simulink model "Top_Model"  (R2020a)
settings: Solver=ode4  StartTime=0.0  StopTime=60  FixedStep=DT  MaxStep=DT  RelTol=1e-3  EnableMultiTasking=on
values from neighbouring files (symbols this model uses):
  OutList = get_OutList(outfile_path)    [run_Top_Model_multi.m]
  tp = turbine_params_5MW()    [baseline_design.m]    (also in run_Top_Model.m)
undefined symbols (not defined in the file or in its folder): strmatch
settings Model: Creator=bjonkman  LastModifiedBy=lpwoolcock
settings SolverCC: AutoInsertRateTranBlk=on
settings DataIOCC: SaveFormat=Array  SignalLoggingSaveFormat=ModelDataLogs  SaveOutput=off  SaveTime=off  ReturnWorkspaceOutputs=off  SignalLoggingName=sigsOut
settings OptimizationCC: ExpressionDepthLimit=2147483647  LifeSpan=inf
settings DebuggingCC: SaveWithParameterizedLinksMsg=none  UnderspecifiedInitializationDetection=Classic  MergeDetectMultiDrivingBlocksExec=none  SignalResolutionControl=TryResolveAllWithWarning  MultiTaskDSMMsg=warning  MultiTaskCondExecSysMsg=none  FcnCallInpInsideContextMsg=warning  StateNameClashWarn=warning  SFUnexpectedBacktrackingDiag=warning  SFNoUnconditionalDefaultTransitionDiag=warning  SFExecutionAtInitializationDiag=none  ArithmeticOperatorsInVariantConditions=warning
settings HardwareCC: ProdBitPerPointer=32  ProdBitPerSizeT=32  ProdBitPerPtrDiffT=32  ProdLargestAtomicFloat=None  ProdIntDivRoundTo=Undefined  ProdEndianess=Unspecified  ProdWordSize=32  ProdHWDeviceType=32-bit Generic  TargetUnknown=on
settings ModelReferenceCC: PropagateSignalLabelsOutOfModel=off
settings SFSimCC: SimUseLocalCustomCode=off  CustomCodeUndefinedFunction=UseInterfaceOnly
settings RTWCC: RTWUseLocalCustomCode=off
settings CodeAppCC: StateflowObjectComments=on
settings GRTTargetCC: TargetLangStandard=C89/C90 (ANSI)  ModelReferenceCompliant=off  ParMdlRefBuildCompliant=off  CompOptLevelCompliant=off  ConcurrentExecutionCompliant=off  CombineOutputUpdateFcns=off  MatFileLogging=off  GRTInterface=on
settings ConfigComp: CovMetricSettings=dw  CovHtmlReporting=on  CovSaveCumulativeToWorkspaceVar=on  CovSaveSingleToWorkspaceVar=on  CovExternalEMLEnable=off

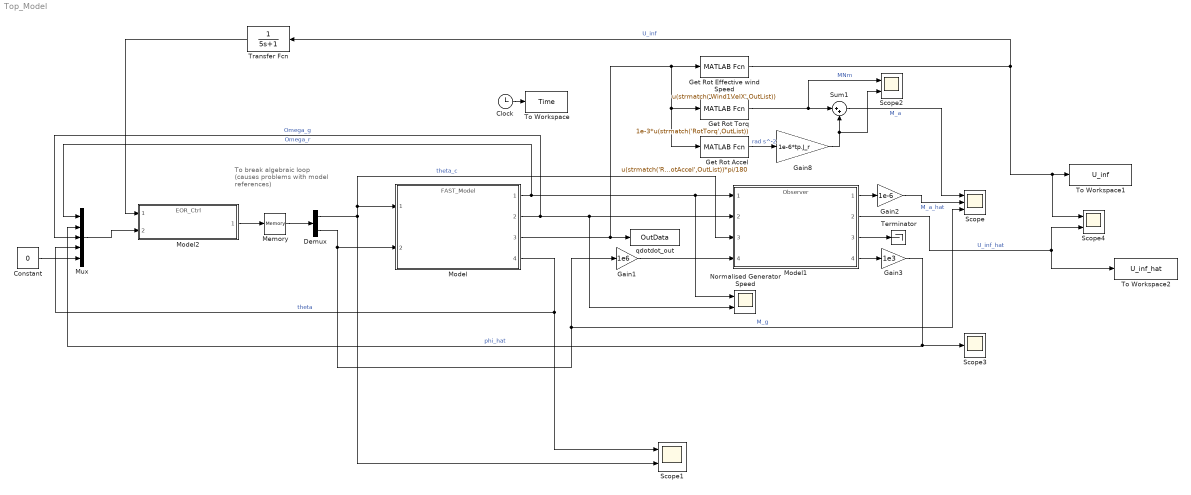
== system Top_Model ==
  note: To break algebraic loop (causes problems with model references)
  Clock : Clock
  Constant : Constant  Value=0
  Demux : Demux  Outputs=2
  Gain1 : Gain  Gain=1e6
  Gain2 : Gain  Gain=1e-6
  Gain3 : Gain  Gain=1e3
  Gain8 : Gain  Gain=1e-6*tp.J_r
  Get Rot Accel : MATLABFcn  MATLABFcn=u(strmatch('RotAccel',OutList))*pi/180
  Get Rot Effective wind Speed : MATLABFcn  MATLABFcn=u(strmatch('Wind1VelX',OutList))
  Get Rot Torq : MATLABFcn  MATLABFcn=1e-3*u(strmatch('RotTorq',OutList))
  Memory : Memory
  Model : ModelReference  ModelNameDialog=FAST_Model.slx  SimulationMode=Normal  ModelReferenceVersion=1.8
  Model1 : ModelReference  ModelNameDialog=Observer.slx  SimulationMode=Normal  ModelReferenceVersion=1.15
  Model2 : ModelReference  ModelNameDialog=EOR_Ctrl.slx  SimulationMode=Normal  ModelReferenceVersion=1.66
  Mux : Mux  Inputs=5
  Normalised Generator Speed : Scope  NumInputPorts=2
  Scope : Scope  NumInputPorts=3
  Scope1 : Scope  NumInputPorts=2
  Scope2 : Scope  NumInputPorts=2
  Scope3 : Scope
  Scope4 : Scope  NumInputPorts=2
  Sum1 : Sum  Inputs=|++
  Terminator : Terminator
  To Workspace : ToWorkspace  VariableName=Time  SampleTime=-1
  To Workspace1 : ToWorkspace  VariableName=U_inf  SaveFormat=Timeseries  SampleTime=-1
  To Workspace2 : ToWorkspace  VariableName=U_inf_hat  SaveFormat=Timeseries  SampleTime=-1
  Transfer Fcn : TransferFcn  Denominator=[5 1]
  qdotdot_out : ToWorkspace  VariableName=OutData  SampleTime=-1
  wires:
  Clock/1 -> To Workspace/1
  Model/3 -> Get Rot Accel/1, Get Rot Torq/1, Get Rot Effective wind Speed/1, qdotdot_out/1
  Get Rot Effective wind Speed/1 -> To Workspace1/1, Scope4/1, Transfer Fcn/1  "U_inf"
  Model1/1 -> Gain2/1
  Get Rot Accel/1 -> Gain8/1  "rad s^-2"
  Get Rot Torq/1 -> Scope2/1, Sum1/1  "MNm"
  Sum1/1 -> Scope/1  "M_a"
  Gain8/1 -> Sum1/2, Scope2/2
  Model/1 -> Mux/1, Normalised Generator Speed/1, Model1/1  "Omega_r"
  Model/2 -> Mux/3, Model1/2, Normalised Generator Speed/2  "Omega_g"
  Model1/3 -> Terminator/1
  Model/4 -> Mux/4, Scope1/1  "theta"
  Model2/1 -> Memory/1
  Memory/1 -> Demux/1
  Mux/1 -> Model2/2
  Model1/4 -> Gain3/1
  Constant/1 -> Mux/5
  Demux/1 -> Model1/3, Model/1, Scope1/2  "theta_c"
  Demux/2 -> Model/2, Gain1/1, Scope/3  "M_g"
  Gain1/1 -> Model1/4
  Gain2/1 -> Scope/2  "M_a_hat"
  Gain3/1 -> Mux/2, Scope3/1  "phi_hat"
  Model1/2 -> Scope4/2, To Workspace2/1  "U_inf_hat"
  Transfer Fcn/1 -> Model2/1
